simulink model "Sim"  (R2018a)
settings: Solver=VariableStepAuto  StartTime=0.0  StopTime=10.0  RelTol=1e-3
values from neighbouring files (symbols this model uses):
  A_imu = [1 0 Ts_imu 0 Ts_imu^2/2 0 ... (first row only)    [GPS_IMU.m]    (also in GPS_IMU_V2.m = [1 0 Ts_imu 0;0 1 0 Ts_imu;0 0 1 0;0 0 0 1])
  B_imu = [Ts_imu^2/2 0;0 Ts_imu^2/2;Ts_imu 0;0 Ts_imu]    [GPS_IMU_V2.m]
  C_imu = [0 0 0 0 1 0;0 0 0 0 0 1]    [GPS_IMU.m]    (also in GPS_IMU_V2.m = [1 0 0 0;0 1 0 0])
  Rv_imu = [0.01 0;0 0.01]    [GPS_IMU.m]
  Rw_imu = 1*[Ts_imu^5/20 0 Ts_imu^4/8 0 Ts_imu^3/6 0 ... (first row only)    [GPS_IMU.m]    (also in GPS_IMU_V2.m = 0.01*diag([Ts_imu^2/2 Ts_imu^2/2 Ts_imu Ts_imu]))
  Ts_imu = 0.02    [GPS_IMU.m]    (also in GPS_IMU_V2.m = 0.01)
settings Model: Creator=marcus  LastModifiedBy=marcus

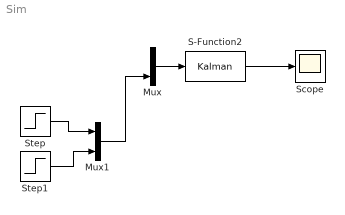
== system Sim ==
  Mux : Mux  Inputs=2
  Mux1 : Mux  Inputs=2
  S-Function2 : S-Function  FunctionName=Kalman  Parameters=Ts_imu,A_imu,B_imu,C_imu,Rw_imu,Rv_imu  SFunctionDeploymentMode=off  EnableBusSupport=off
  Scope : Scope
  Step : Step  SampleTime=0
  Step1 : Step  Time=2  SampleTime=0
  wires:
  Mux/1 -> S-Function2/1
  Step/1 -> Mux1/1
  Step1/1 -> Mux1/2
  Mux1/1 -> Mux/2
  S-Function2/1 -> Scope/1
